simulink model "quadrotor_adrc_controller"  (R2015a)
settings: Solver=ode45  StartTime=0.0  StopTime=15  RelTol=1e-3
values from neighbouring files (symbols this model uses):
  k1p = u(5)    [quadrotor_adrc_controller.m]
  k2p = u(6)    [quadrotor_adrc_controller.m]
  kdx = u(14)    [quadrotor_adrc_controller.m]
  kdy = u(16)    [quadrotor_adrc_controller.m]
  kpx = u(13)    [quadrotor_adrc_controller.m]
  kpy = u(15)    [quadrotor_adrc_controller.m]
undefined symbols (not defined in the file or in its folder): k1k, k1t, k1z, k2k, k2t, k2z
settings Model: Creator=kbmaj  LastModifiedBy=kbmaj

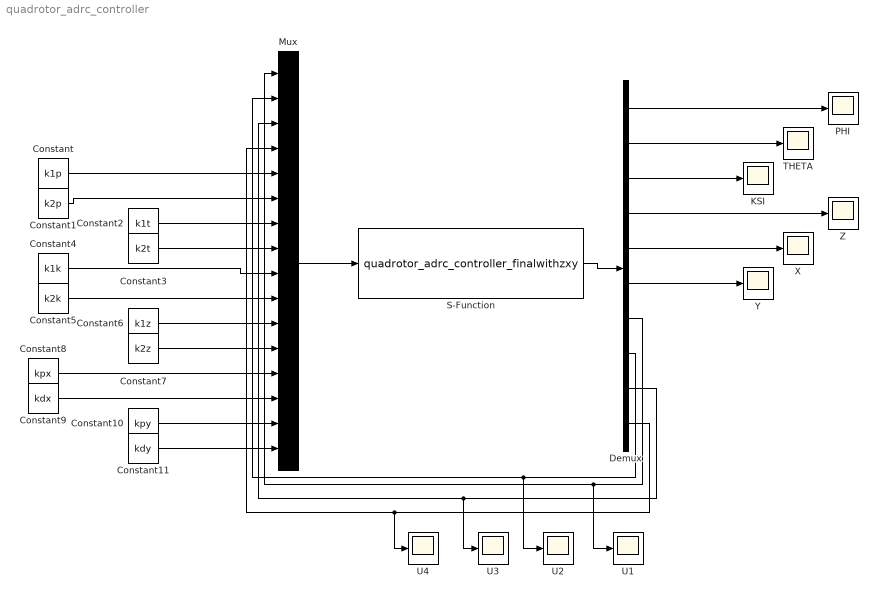
== system quadrotor_adrc_controller ==
  Constant : Constant  Value=k1p
  Constant1 : Constant  Value=k2p
  Constant10 : Constant  Value=kpy
  Constant11 : Constant  Value=kdy
  Constant2 : Constant  Value=k1t
  Constant3 : Constant  Value=k2t
  Constant4 : Constant  Value=k1k
  Constant5 : Constant  Value=k2k
  Constant6 : Constant  Value=k1z
  Constant7 : Constant  Value=k2z
  Constant8 : Constant  Value=kpx
  Constant9 : Constant  Value=kdx
  Demux : Demux  Outputs=10
  KSI : Scope
  Mux : Mux  Inputs=16
  PHI : Scope
      settings: YMin=-31000  YMax=-22500  SaveName=ScopeData2
  S-Function : S-Function  FunctionName=quadrotor_adrc_controller_finalwithzxy
  THETA : Scope
      settings: YMin=89  YMax=102
  U{1..4} (4 alike) : Scope
      U1 settings: SaveName=ScopeData6
      U2 settings: SaveName=ScopeData7
      U3 settings: SaveName=ScopeData8
      U4 settings: SaveName=ScopeData9
  X : Scope
      settings: SaveName=ScopeData4
  Y : Scope
      settings: YMin=0  YMax=27.5  SaveName=ScopeData5
  Z : Scope
      settings: YMin=415  YMax=467.5  SaveName=ScopeData3
  wires:
  Mux/1 -> S-Function/1
  S-Function/1 -> Demux/1
  Demux/3 -> KSI/1
  Demux/2 -> THETA/1
  Demux/1 -> PHI/1
  Constant/1 -> Mux/5
  Constant1/1 -> Mux/6
  Constant2/1 -> Mux/7
  Constant3/1 -> Mux/8
  Constant4/1 -> Mux/9
  Constant5/1 -> Mux/10
  Constant6/1 -> Mux/11
  Constant7/1 -> Mux/12
  Constant8/1 -> Mux/13
  Constant9/1 -> Mux/14
  Constant10/1 -> Mux/15
  Constant11/1 -> Mux/16
  Demux/4 -> Z/1
  Demux/5 -> X/1
  Demux/6 -> Y/1
  Demux/7 -> U1/1, Mux/1
  Demux/8 -> Mux/2, U2/1
  Demux/9 -> U3/1, Mux/3
  Demux/10 -> U4/1, Mux/4
